simulink model "DiagramaBloques"  (R2014a)
settings: Solver=ode45  StartTime=0.0  StopTime=periodo  RelTol=1e-3
PreLoadFcn:
  | variables
InitFcn:
  | eval('variables');
  | variables
StartFcn:
  | variables
values from neighbouring files (symbols this model uses):
  C = 0.6e-6    (= 6e-07)    [Circuito_RC.m]    (also in variables.m = 3e-08)
  E = 5    [Circuito_RC.m]    (also in variables.m)
  frecuencia = 935.5    [Circuito_RC.m]    (also in variables.m = 935.9)
  L = 2.37e-3    (= 0.00237)    [Circuito_RC.m]    (also in variables.m)
  R = 10e3    (= 10000)    [Circuito_RC.m]    (also in variables.m)
  Rc = 100    [Circuito_RC.m]    (also in variables.m)
  Rf = 50    [Circuito_RC.m]    (also in variables.m)
  Rl = 0.8    [Circuito_RC.m]    (also in variables.m)
  Rml = 100    [Circuito_RC.m]    (also in variables.m)
settings Model: Creator=jhoan  LastModifiedBy=jhoan

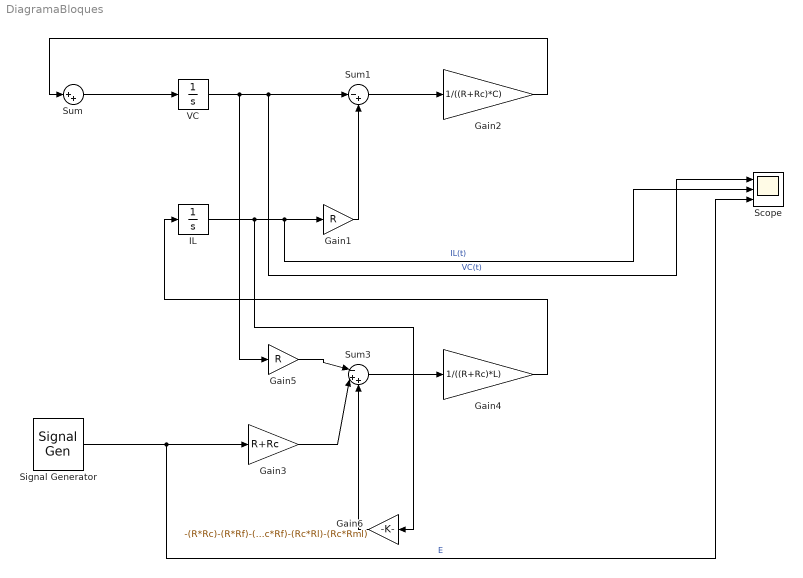
== system DiagramaBloques ==
  Gain1 : Gain  Gain=R
  Gain2 : Gain  Gain=1/((R+Rc)*C)
  Gain3 : Gain  Gain=R+Rc
  Gain4 : Gain  Gain=1/((R+Rc)*L)
  Gain5 : Gain  Gain=R
  Gain6 : Gain  Gain=-(R*Rc)-(R*Rf)-(R*Rl)-(R*Rml)-(Rc*Rf)-(Rc*Rl)-(Rc*Rml)
  IL : Integrator
  Scope : Scope  NumInputPorts=3
      settings: YMin=-5~-5~-5  YMax=5~5~5  SaveName=subSimulink
  Signal Generator : SignalGenerator  WaveForm=square  Amplitude=E  Frequency=frecuencia
  Sum : Sum  Inputs=|++
  Sum1 : Sum  Inputs=|-+
  Sum3 : Sum  Inputs=|-++
  VC : Integrator
  wires:
  Sum/1 -> VC/1
  IL/1 -> Gain6/1, Scope/2, Gain1/1  "IL(t)"
  VC/1 -> Gain5/1, Scope/1, Sum1/1  "VC(t)"
  Gain1/1 -> Sum1/2
  Sum1/1 -> Gain2/1
  Gain2/1 -> Sum/1
  Signal Generator/1 -> Scope/3, Gain3/1  "E"
  Gain3/1 -> Sum3/2
  Sum3/1 -> Gain4/1
  Gain5/1 -> Sum3/1
  Gain4/1 -> IL/1
  Gain6/1 -> Sum3/3
